simulink model "quadrotor_stage3"  (R2026a)
settings: Solver=ode4  StartTime=0  StopTime=18  FixedStep=0.005  MaxStep=0.005  RelTol=1e-6
undefined symbols (not defined in the file): DiscIntNeverNeededParam
settings Model: Creator=ASUS  LastModifiedBy=ASUS

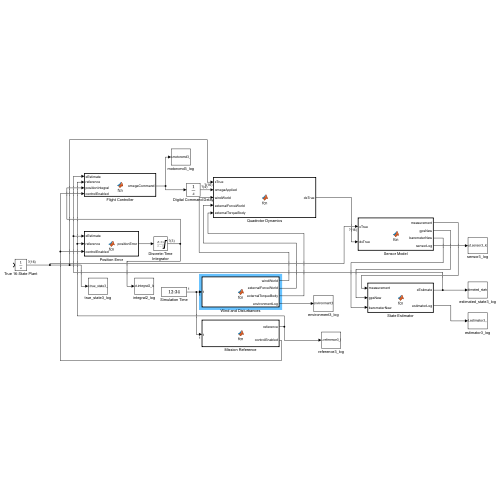
[thumbnail: Simulink's stored preview of the top-level diagram]
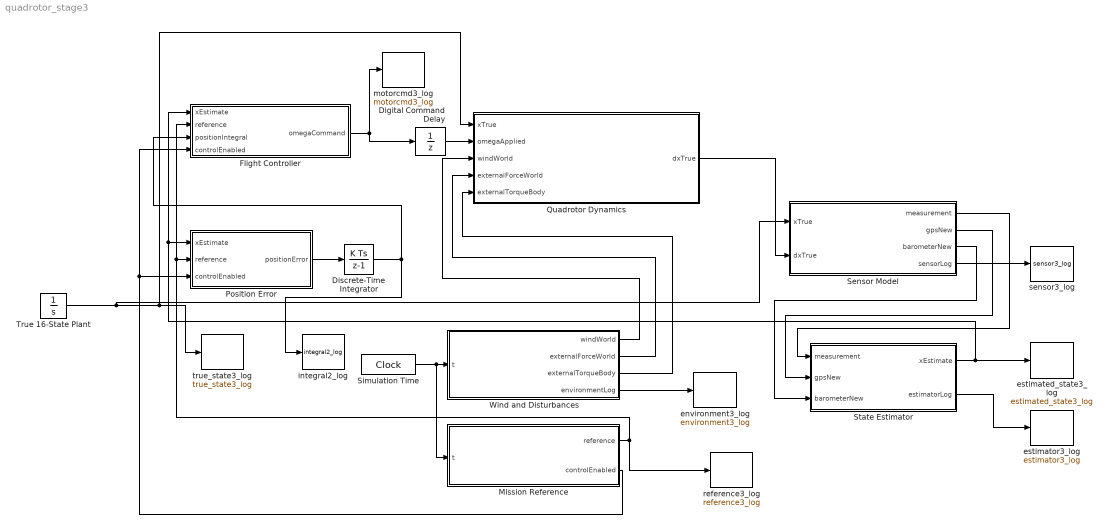
== system quadrotor_stage3 ==
  Digital Command Delay : UnitDelay  InitialCondition=sqrt(1.20*9.81/(4*1.8e-5))*ones(4,1)  SampleTime=0.005
  Discrete-Time Integrator : DiscreteIntegrator  InitialCondition=zeros(3,1)  SampleTime=0.005  LimitOutput=on  UpperSaturationLimit=[4;4;1.5]  LowerSaturationLimit=[-4;-4;-1.5]  ICPrevOutput=DiscIntNeverNeededParam  ICPrevScaledInput=DiscIntNeverNeededParam
  Flight Controller : MATLAB Function  TreatAsAtomicUnit=on
  Mission Reference : MATLAB Function  TreatAsAtomicUnit=on
  Position Error : MATLAB Function  TreatAsAtomicUnit=on
  Quadrotor Dynamics : MATLAB Function  TreatAsAtomicUnit=on
  Sensor Model : MATLAB Function  TreatAsAtomicUnit=on
  Simulation Time : DigitalClock
  State Estimator : MATLAB Function  TreatAsAtomicUnit=on
  True 16-State Plant : Integrator  InitialCondition=[zeros(12,1); sqrt(1.20*9.81/(4*1.8e-5))*ones(4,1)]
  Wind and Disturbances : MATLAB Function  TreatAsAtomicUnit=on
  environment3_log : ToWorkspace  VariableName=environment3_log  SaveFormat=Timeseries  SampleTime=-1
      settings: Save2DSignal=2-D array (concatenate along first dimension)
  estimated_state3_log : ToWorkspace  VariableName=estimated_state3_log  SaveFormat=Timeseries  SampleTime=-1
      settings: Save2DSignal=2-D array (concatenate along first dimension)
  estimator3_log : ToWorkspace  VariableName=estimator3_log  SaveFormat=Timeseries  SampleTime=-1
      settings: Save2DSignal=2-D array (concatenate along first dimension)
  integral2_log : ToWorkspace  VariableName=integral2_log  SaveFormat=Timeseries  SampleTime=-1
      settings: Save2DSignal=2-D array (concatenate along first dimension)
  motorcmd3_log : ToWorkspace  VariableName=motorcmd3_log  SaveFormat=Timeseries  SampleTime=-1
      settings: Save2DSignal=2-D array (concatenate along first dimension)
  reference3_log : ToWorkspace  VariableName=reference3_log  SaveFormat=Timeseries  SampleTime=-1
      settings: Save2DSignal=2-D array (concatenate along first dimension)
  sensor3_log : ToWorkspace  VariableName=sensor3_log  SaveFormat=Timeseries  SampleTime=-1
      settings: Save2DSignal=2-D array (concatenate along first dimension)
  true_state3_log : ToWorkspace  VariableName=true_state3_log  SaveFormat=Timeseries  SampleTime=-1
      settings: Save2DSignal=2-D array (concatenate along first dimension)
  wires:
  Flight Controller/1(omegaCommand) -> Digital Command Delay/1, motorcmd3_log/1
  True 16-State Plant/1 -> Sensor Model/1(xTrue), true_state3_log/1, Quadrotor Dynamics/1(xTrue)
  Position Error/1(positionError) -> Discrete-Time Integrator/1
  Discrete-Time Integrator/1 -> integral2_log/1, Flight Controller/3(positionIntegral)
  Simulation Time/1 -> Mission Reference/1(t), Wind and Disturbances/1(t)
  Wind and Disturbances/1(windWorld) -> Quadrotor Dynamics/3(windWorld)
  Wind and Disturbances/2(externalForceWorld) -> Quadrotor Dynamics/4(externalForceWorld)
  Wind and Disturbances/3(externalTorqueBody) -> Quadrotor Dynamics/5(externalTorqueBody)
  Wind and Disturbances/4(environmentLog) -> environment3_log/1
  Quadrotor Dynamics/1(dxTrue) -> Sensor Model/2(dxTrue)
  Sensor Model/1(measurement) -> State Estimator/1(measurement)
  Sensor Model/2(gpsNew) -> State Estimator/2(gpsNew)
  Sensor Model/3(barometerNew) -> State Estimator/3(barometerNew)
  State Estimator/1(xEstimate) -> estimated_state3_log/1, Position Error/1(xEstimate), Flight Controller/1(xEstimate)
  Mission Reference/1(reference) -> reference3_log/1, Position Error/2(reference), Flight Controller/2(reference)
  Mission Reference/2(controlEnabled) -> Position Error/3(controlEnabled), Flight Controller/4(controlEnabled)
  Digital Command Delay/1 -> Quadrotor Dynamics/2(omegaApplied)
  State Estimator/2(estimatorLog) -> estimator3_log/1
  Sensor Model/4(sensorLog) -> sensor3_log/1

== matlab function quadrotor_stage3/Quadrotor Dynamics ==
  data: xTrue input; dxTrue output; omegaApplied input; windWorld input; externalForceWorld input; externalTorqueBody input
function dxTrue = fcn(xTrue, omegaApplied, windWorld, ...
    externalForceWorld, externalTorqueBody)
%#codegen
dxTrue = quadDynamicsStage3(xTrue, omegaApplied, windWorld, ...
    externalForceWorld, externalTorqueBody);
end

== matlab function quadrotor_stage3/Flight Controller ==
  settings: updateMethod=DISCRETE  sampleTime=0.005
  data: xEstimate input; omegaCommand output; reference input; positionIntegral input; controlEnabled input
function omegaCommand = fcn(xEstimate, reference, ...
    positionIntegral, controlEnabled)
%#codegen
omegaCommand = flightControllerStage3(xEstimate, reference, ...
    positionIntegral, controlEnabled);
end

== matlab function quadrotor_stage3/Position Error ==
  settings: updateMethod=DISCRETE  sampleTime=0.005
  data: xEstimate input; positionError output; reference input; controlEnabled input
function positionError = fcn(xEstimate, reference, controlEnabled)
%#codegen
positionError = positionErrorStage3( ...
    xEstimate, reference, controlEnabled);
end

== matlab function quadrotor_stage3/Wind and Disturbances ==
  data: t input; windWorld output; externalForceWorld output; externalTorqueBody output; environmentLog output
function [windWorld, externalForceWorld, ...
    externalTorqueBody, environmentLog] = fcn(t)
%#codegen
[windWorld, externalForceWorld, externalTorqueBody, environmentLog] = ...
    environmentStage3(t);
end

== matlab function quadrotor_stage3/Mission Reference ==
  data: t input; reference output; controlEnabled output
function [reference, controlEnabled] = fcn(t)
%#codegen
[reference, controlEnabled] = missionReferenceStage3(t);
end

== matlab function quadrotor_stage3/Sensor Model ==
  settings: updateMethod=DISCRETE  sampleTime=0.005
  data: xTrue input; measurement output; dxTrue input; gpsNew output; barometerNew output; sensorLog output
function [measurement, gpsNew, barometerNew, sensorLog] = ...
    fcn(xTrue, dxTrue)
%#codegen
[measurement, gpsNew, barometerNew, sensorLog] = ...
    sensorModelStage3(xTrue, dxTrue);
end

== matlab function quadrotor_stage3/State Estimator ==
  settings: updateMethod=DISCRETE  sampleTime=0.005
  data: measurement input; xEstimate output; gpsNew input; barometerNew input; estimatorLog output
function [xEstimate, estimatorLog] = ...
    fcn(measurement, gpsNew, barometerNew)
%#codegen

[xEstimate, estimatorLog] = stateEstimatorStage3( ...
    measurement, gpsNew, barometerNew);
end
